simulink model "Test_Schnittstelle"  (R2018a)
settings: Solver=FixedStepAuto  StartTime=0.0  StopTime=inf  FixedStep=0.0000001  RelTol=1e-3
model workspace (MAT data in the model file):
  Address = Simulink.Signal
  Address.DataType = 'double'
  Address.Dimensions = 1
  Address.DimensionsMode = 'Fixed'
  Address.Complexity = 'real'
  Address.SampleTime = -1
  Address.SamplingMode = 'auto'
  Address.InitialValue = '0'
  De_1 = Simulink.Signal
  De_1.DataType = 'double'
  De_1.Dimensions = 1
  De_1.DimensionsMode = 'Fixed'
  De_1.Complexity = 'real'
  De_1.SampleTime = -1
  De_1.SamplingMode = 'auto'
  De_1.InitialValue = '0'
  De_2 = Simulink.Signal
  De_2.DataType = 'double'
  De_2.Dimensions = 1
  De_2.DimensionsMode = 'Fixed'
  De_2.Complexity = 'real'
  De_2.SampleTime = -1
  De_2.SamplingMode = 'auto'
  De_sum_1 = Simulink.Signal
  De_sum_1.DataType = 'double'
  De_sum_1.Dimensions = -1
  De_sum_1.DimensionsMode = 'Fixed'
  De_sum_1.Complexity = 'real'
  De_sum_1.SampleTime = -1
  De_sum_1.SamplingMode = 'auto'
  De_sum_1.InitialValue = '0'
  De_sum_2 = Simulink.Signal
  De_sum_2.DataType = 'double'
  De_sum_2.Dimensions = -1
  De_sum_2.DimensionsMode = 'Fixed'
  De_sum_2.Complexity = 'real'
  De_sum_2.SampleTime = -1
  De_sum_2.SamplingMode = 'auto'
  De_sum_2.InitialValue = '0'
  Filter = Simulink.Signal
  Filter.DataType = 'double'
  Filter.Dimensions = [20 7]
  Filter.DimensionsMode = 'Fixed'
  Filter.Complexity = 'real'
  Filter.SampleTime = -1
  Filter.SamplingMode = 'auto'
  Filter.InitialValue = 'zeros(20,7)'
  Handshake_1 = Simulink.Signal
  Handshake_1.DataType = 'boolean'
  Handshake_1.Dimensions = -1
  Handshake_1.DimensionsMode = 'Fixed'
  Handshake_1.Complexity = 'real'
  Handshake_1.SampleTime = -1
  Handshake_1.SamplingMode = 'auto'
  Handshake_1.InitialValue = 'false'
  Handshake_2 = Simulink.Signal
  Handshake_2.DataType = 'boolean'
  Handshake_2.Dimensions = -1
  Handshake_2.DimensionsMode = 'Fixed'
  Handshake_2.Complexity = 'real'
  Handshake_2.SampleTime = -1
  Handshake_2.SamplingMode = 'auto'
  Handshake_2.InitialValue = 'false'
  Recv_Buffer = Simulink.Signal
  Recv_Buffer.DataType = 'double'
  Recv_Buffer.Dimensions = [20 7]
  Recv_Buffer.DimensionsMode = 'Fixed'
  Recv_Buffer.Complexity = 'real'
  Recv_Buffer.SampleTime = -1
  Recv_Buffer.SamplingMode = 'auto'
  Recv_Buffer.InitialValue = 'zeros(20,7)'
  Send_Buffer_1 = Simulink.Signal
  Send_Buffer_1.DataType = 'double'
  Send_Buffer_1.Dimensions = [1 100]
  Send_Buffer_1.DimensionsMode = 'Fixed'
  Send_Buffer_1.Complexity = 'real'
  Send_Buffer_1.SampleTime = -1
  Send_Buffer_1.SamplingMode = 'auto'
  Send_Buffer_1.InitialValue = '[101, 102, zeros(1,98)]'
  Send_Buffer_2 = Simulink.Signal
  Send_Buffer_2.DataType = 'double'
  Send_Buffer_2.Dimensions = [1 100]
  Send_Buffer_2.DimensionsMode = 'Fixed'
  Send_Buffer_2.Complexity = 'real'
  Send_Buffer_2.SampleTime = -1
  Send_Buffer_2.SamplingMode = 'auto'
  Send_Buffer_2.InitialValue = '[101, 102, zeros(1,98)]'
  T_recv_1 = Simulink.Signal
  T_recv_1.DataType = 'double'
  T_recv_1.Dimensions = 1
  T_recv_1.DimensionsMode = 'Fixed'
  T_recv_1.Complexity = 'real'
  T_recv_1.SampleTime = -1
  T_recv_1.SamplingMode = 'auto'
  T_recv_1.InitialValue = '0'
  T_recv_2 = Simulink.Signal
  T_recv_2.DataType = 'auto'
  T_recv_2.Dimensions = 1
  T_recv_2.DimensionsMode = 'Fixed'
  T_recv_2.Complexity = 'real'
  T_recv_2.SampleTime = -1
  T_recv_2.SamplingMode = 'auto'
  T_recv_2.InitialValue = '0'
  T_send_1 = Simulink.Signal
  T_send_1.DataType = 'double'
  T_send_1.Dimensions = 1
  T_send_1.DimensionsMode = 'Fixed'
  T_send_1.Complexity = 'real'
  T_send_1.SampleTime = -1
  T_send_1.SamplingMode = 'auto'
  T_send_1.InitialValue = '0'
  T_send_2 = Simulink.Signal
  T_send_2.DataType = 'double1'
  T_send_2.Dimensions = 1
  T_send_2.DimensionsMode = 'Fixed'
  T_send_2.Complexity = 'real'
  T_send_2.SampleTime = -1
  T_send_2.SamplingMode = 'auto'
(part 1 of 2)
settings Model: Creator=张紫薇  LastModifiedBy=lenovo

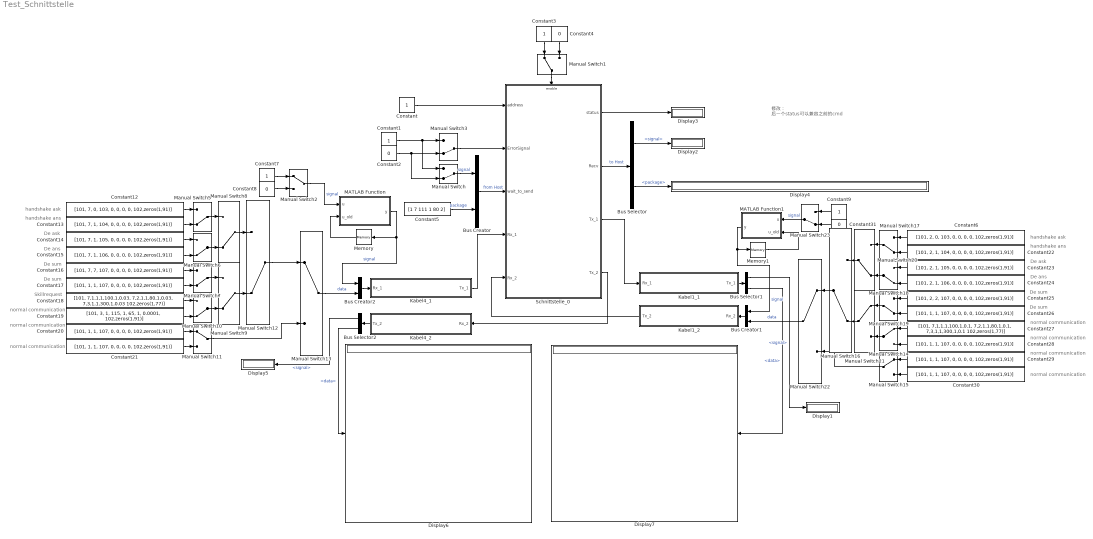
== system Test_Schnittstelle ==
  note: 修改：
      | 后一个status可以兼容之前的cmd
  note: handshake ask
  note: handshake ans
  note: De ask
  note: De ans
  note: De sum
  note: De sum
  note: Skillrequest
  note: normal communication
  note: normal communication
  note: normal communication
  note: normal communication
  note: normal communication
  note: handshake ask
  note: normal communication
  note: De sum
  note: handshake ans
  note: normal communication
  note: De ans
  note: De ask
  note: De sum
  Bus Creator : BusCreator  Inputs=2
  Bus Creator1 : BusCreator  Inputs=2
  Bus Creator2 : BusCreator  Inputs=2
  Bus Selector : BusSelector  OutputSignals=signal,package
  Bus Selector1 : BusSelector  OutputSignals=signal,data
  Bus Selector2 : BusSelector  OutputSignals=signal,data
  Constant : Constant  OutDataTypeStr=double
  Constant{1,3,7,9} (4 alike) : Constant  OutDataTypeStr=boolean
  Constant12 : Constant  Value=[101, 7, 0, 103, 0, 0, 0, 0, 102,zeros(1,91)]  OutDataTypeStr=double
  Constant13 : Constant  Value=[101, 7, 1, 104, 0, 0, 0, 0, 102,zeros(1,91)]  OutDataTypeStr=double
  Constant14 : Constant  Value=[101, 7, 1, 105, 0, 0, 0, 0, 102,zeros(1,91)]  OutDataTypeStr=double
  Constant15 : Constant  Value=[101, 7, 1, 106, 0, 0, 0, 0, 102,zeros(1,91)]  OutDataTypeStr=double
  Constant16 : Constant  Value=[101, 7, 7, 107, 0, 0, 0, 0, 102,zeros(1,91)]  OutDataTypeStr=double
  Constant{17,20..21,26,28..30} (7 alike) : Constant  Value=[101, 1, 1, 107, 0, 0, 0, 0, 102,zeros(1,91)]  OutDataTypeStr=double
  Constant18 : Constant  Value=[101, 7,1,1,1,100,1,0.03, 7,2,1,1,80,1,0.03, 7,3,1,1,300,1,0.03 102,zeros(1,77)]  OutDataTypeStr=double
  Constant19 : Constant  Value=[101, 3, 1, 115, 1, 65, 1, 0.0001, 102,zeros(1,91)]  OutDataTypeStr=double
  Constant{2,4,8,31} (4 alike) : Constant  Value=0  OutDataTypeStr=boolean
  Constant22 : Constant  Value=[101, 2, 1, 104, 0, 0, 0, 0, 102,zeros(1,91)]  OutDataTypeStr=double
  Constant23 : Constant  Value=[101, 2, 1, 105, 0, 0, 0, 0, 102,zeros(1,91)]  OutDataTypeStr=double
  Constant24 : Constant  Value=[101, 2, 1, 106, 0, 0, 0, 0, 102,zeros(1,91)]  OutDataTypeStr=double
  Constant25 : Constant  Value=[101, 2, 2, 107, 0, 0, 0, 0, 102,zeros(1,91)]  OutDataTypeStr=double
  Constant27 : Constant  Value=[101, 7,1,1,1,100,1,0.1, 7,2,1,1,80,1,0.1, 7,3,1,1,300,1,0.1 102,zeros(1,77)]  OutDataTypeStr=double
  Constant5 : Constant  Value=[1 7 111 1 80 2]  OutDataTypeStr=double
  Constant6 : Constant  Value=[101, 2, 0, 103, 0, 0, 0, 0, 102,zeros(1,91)]  OutDataTypeStr=double
  Display{1..7} (7 alike) : Display
      Display4 settings: Decimation=7
  Kabel1_1 : Subsystem  TreatAsAtomicUnit=on
  Kabel1_2 : Subsystem  TreatAsAtomicUnit=on
  Kabel4_1 : Subsystem  TreatAsAtomicUnit=on
  Kabel4_2 : Subsystem  TreatAsAtomicUnit=on
  MATLAB Function : MATLAB Function  TreatAsAtomicUnit=on  SystemSampleTime=0.00001
  MATLAB Function1 : MATLAB Function  TreatAsAtomicUnit=on  SystemSampleTime=0.00001
  Manual Switch{,3,5..10,12,16..20,23} (15 alike) : ManualSwitch  CurrentSetting=0
  Manual Switch{1..2,11,13..15,21..22} (8 alike) : ManualSwitch
  Memory : Memory  InitialCondition=false
  Memory1 : Memory  InitialCondition=false
  Schnittstelle_0 : Subsystem
  wires:
  Kabel4_2/1(Tx_2) -> Bus Selector2/1
  Bus Creator1/1 -> Kabel1_2/1(Rx_2)
  Bus Selector2/1 -> Display5/1  "<signal>"
  Bus Creator/1 -> Schnittstelle_0/3(wait_to_send)  "from Host"
  Constant8/1 -> Manual Switch2/2
  Kabel4_1/1(Tx_1) -> Schnittstelle_0/4(Rx_1)
  Manual Switch/1 -> Bus Creator/1  "signal"
  Bus Selector/1 -> Display2/1  "<signal>"
  Kabel1_1/1(Tx_1) -> Bus Selector1/1
  Manual Switch3/1 -> Schnittstelle_0/2(ErrorSignal)
  Bus Selector/2 -> Display4/1  "<package>"
  Manual Switch13/1 -> Bus Creator2/2  "data"
  MATLAB Function/1(y) -> Bus Creator2/1, Memory/1  "signal"
  Constant5/1 -> Bus Creator/2  "package"
  Constant7/1 -> Manual Switch2/1
  Kabel1_2/1(Tx_2) -> Schnittstelle_0/5(Rx_2)
  Constant4/1 -> Manual Switch1/2
  Constant1/1 -> Manual Switch/1, Manual Switch3/1
  Constant3/1 -> Manual Switch1/1
  Constant/1 -> Schnittstelle_0/1(address)
  MATLAB Function1/1(y) -> Bus Creator1/1, Memory1/1  "signal"
  Bus Selector1/1 -> Display1/1  "<signal>"
  Bus Creator2/1 -> Kabel4_1/1(Rx_1)
  Schnittstelle_0/1(status) -> Display3/1
  Bus Selector1/2 -> Display7/1  "<data>"
  Schnittstelle_0/4(Tx_2) -> Kabel4_2/1(Rx_2)
  Manual Switch1/1 -> Schnittstelle_0/Enable
  Constant2/1 -> Manual Switch/2, Manual Switch3/2
  Bus Selector2/2 -> Display6/1  "<data>"
  Schnittstelle_0/2(Recv) -> Bus Selector/1  "to Host"
  Schnittstelle_0/3(Tx_1) -> Kabel1_1/1(Rx_1)
  Constant12/1 -> Manual Switch5/1
  Constant13/1 -> Manual Switch5/2
  Constant14/1 -> Manual Switch6/1
  Constant15/1 -> Manual Switch6/2
  Constant16/1 -> Manual Switch7/1
  Constant17/1 -> Manual Switch7/2
  Manual Switch5/1 -> Manual Switch8/1
  Manual Switch6/1 -> Manual Switch8/2
  Manual Switch7/1 -> Manual Switch9/1
  Manual Switch10/1 -> Manual Switch9/2
  Constant18/1 -> Manual Switch10/1
  Constant19/1 -> Manual Switch10/2
  Constant20/1 -> Manual Switch11/1
  Constant21/1 -> Manual Switch11/2
  Manual Switch9/1 -> Manual Switch12/2
  Manual Switch8/1 -> Manual Switch12/1
  Manual Switch12/1 -> Manual Switch13/1
  Manual Switch11/1 -> Manual Switch13/2
  Constant6/1 -> Manual Switch17/1
  Constant22/1 -> Manual Switch17/2
  Constant23/1 -> Manual Switch18/1
  Constant24/1 -> Manual Switch18/2
  Constant25/1 -> Manual Switch19/1
  Constant26/1 -> Manual Switch19/2
  Constant27/1 -> Manual Switch14/1
  Constant28/1 -> Manual Switch14/2
  Constant29/1 -> Manual Switch15/1
  Constant30/1 -> Manual Switch15/2
  Manual Switch17/1 -> Manual Switch20/1
  Manual Switch18/1 -> Manual Switch20/2
  Manual Switch19/1 -> Manual Switch21/1
  Manual Switch14/1 -> Manual Switch21/2
  Manual Switch20/1 -> Manual Switch16/1
  Manual Switch21/1 -> Manual Switch16/2
  Manual Switch15/1 -> Manual Switch22/2
  Manual Switch22/1 -> Bus Creator1/2  "data"
  Manual Switch16/1 -> Manual Switch22/1
  Manual Switch2/1 -> MATLAB Function/1(u)  "signal"
  Memory/1 -> MATLAB Function/2(u_old)
  Memory1/1 -> MATLAB Function1/2(u_old)
  Manual Switch23/1 -> MATLAB Function1/1(u)  "signal"
  Constant9/1 -> Manual Switch23/1
  Constant31/1 -> Manual Switch23/2

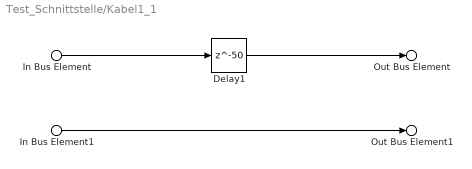
== system Test_Schnittstelle/Kabel1_1 ==
  In Bus Element : Inport  PortName=Rx_1  Element=signal
  In Bus Element1 : Inport  PortName=Rx_1  Element=data
  Delay1 : Delay  DelayLength=50
  Out Bus Element : Outport  PortName=Tx_1  Element=signal
  Out Bus Element1 : Outport  PortName=Tx_1  Element=data
  wires:
  In Bus Element/1 -> Delay1/1
  Delay1/1 -> Out Bus Element/1
  In Bus Element1/1 -> Out Bus Element1/1

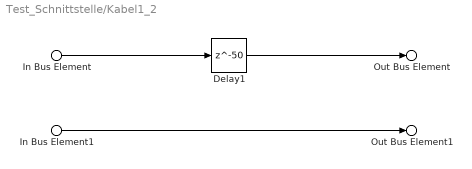
== system Test_Schnittstelle/Kabel1_2 ==
  In Bus Element : Inport  PortName=Rx_2  Element=signal
  In Bus Element1 : Inport  PortName=Rx_2  Element=data
  Delay1 : Delay  DelayLength=50
  Out Bus Element : Outport  PortName=Tx_2  Element=signal
  Out Bus Element1 : Outport  PortName=Tx_2  Element=data
  wires:
  In Bus Element/1 -> Delay1/1
  Delay1/1 -> Out Bus Element/1
  In Bus Element1/1 -> Out Bus Element1/1

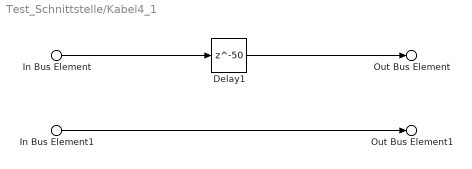
== system Test_Schnittstelle/Kabel4_1 ==
  In Bus Element : Inport  PortName=Rx_1  Element=signal
  In Bus Element1 : Inport  PortName=Rx_1  Element=data
  Delay1 : Delay  DelayLength=50
  Out Bus Element : Outport  PortName=Tx_1  Element=signal
  Out Bus Element1 : Outport  PortName=Tx_1  Element=data
  wires:
  In Bus Element/1 -> Delay1/1
  Delay1/1 -> Out Bus Element/1
  In Bus Element1/1 -> Out Bus Element1/1

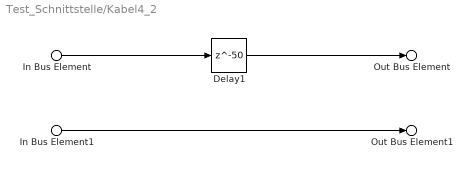
== system Test_Schnittstelle/Kabel4_2 ==
  In Bus Element : Inport  PortName=Rx_2  Element=signal
  In Bus Element1 : Inport  PortName=Rx_2  Element=data
  Delay1 : Delay  DelayLength=50
  Out Bus Element : Outport  PortName=Tx_2  Element=signal
  Out Bus Element1 : Outport  PortName=Tx_2  Element=data
  wires:
  In Bus Element/1 -> Delay1/1
  Delay1/1 -> Out Bus Element/1
  In Bus Element1/1 -> Out Bus Element1/1

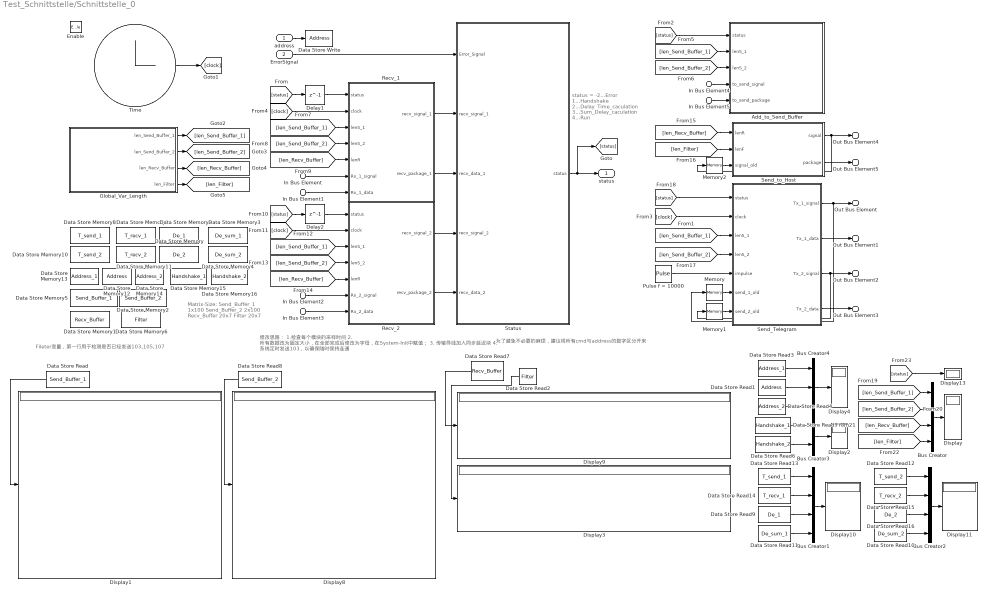
== system Test_Schnittstelle/Schnittstelle_0 ==
  note: 为了避免不必要的麻烦，建议将所有cmd与address的数字区分开来
  note: Fileter变量，第一行用于检测是否已经发送103,105,107
  note: 修改思路：
      | 1.检查每个模块的采样时间
      | 2. 所有数据改为固定大小，在全部完成后修改为字母，在System-Init中赋值；
      | 3. 传输导线加入同步延迟块
      | 4. 系统定时发送103，以确保随时保持连通
  note: status =
      | -2...Error
      |  1...Handshake
      |  2...Delay_Time_caculation
      |  3...Sum_Delay_caculation
      |  4...Run
  note: Matrix-Size:
      | Send_Buffer_1	1x100
      | Send_Buffer_2	2x100
      | Recv_Buffer		20x7
      | Filter			20x7
  address : Inport
  ErrorSignal : Inport  Port=2
  In Bus Element4 : Inport  Port=3  PortName=wait_to_send  Element=signal
  In Bus Element5 : Inport  Port=3  PortName=wait_to_send  Element=package
  In Bus Element : Inport  Port=4  PortName=Rx_1  Element=signal
  In Bus Element1 : Inport  Port=4  PortName=Rx_1  Element=data
  In Bus Element2 : Inport  Port=5  PortName=Rx_2  Element=signal
  In Bus Element3 : Inport  Port=5  PortName=Rx_2  Element=data
  Enable : EnablePort
  Add_to_Send_Buffer : MATLAB Function  TreatAsAtomicUnit=on  SystemSampleTime=0.00001
  Bus Creator : BusCreator  Inputs=4
  Bus Creator1 : BusCreator  Inputs=4
  Bus Creator2 : BusCreator  Inputs=4
  Bus Creator3 : BusCreator  Inputs=2
  Bus Creator4 : BusCreator  Inputs=3
  Data Store Memory : DataStoreMemory  DataStoreName=De_2  ReadBeforeWriteMsg=warning  WriteAfterWriteMsg=warning  WriteAfterReadMsg=warning  ShowAdditionalParam=off  OutDataTypeStr=double  Dimensions=1
  Data Store Memory1 : DataStoreMemory  DataStoreName=Recv_Buffer  ReadBeforeWriteMsg=warning  WriteAfterWriteMsg=warning  WriteAfterReadMsg=warning  InitialValue=zeros(20,7)  VectorParams1D=off  ShowAdditionalParam=off  OutDataTypeStr=double  Dimensions=[20,7]
  Data Store Memory10 : DataStoreMemory  DataStoreName=T_send_2  ReadBeforeWriteMsg=warning  WriteAfterWriteMsg=warning  WriteAfterReadMsg=warning  ShowAdditionalParam=off  OutDataTypeStr=double  Dimensions=1
  Data Store Memory11 : DataStoreMemory  DataStoreName=T_recv_2  ReadBeforeWriteMsg=warning  WriteAfterWriteMsg=warning  WriteAfterReadMsg=warning  ShowAdditionalParam=off  OutDataTypeStr=double  Dimensions=1
  Data Store Memory12 : DataStoreMemory  DataStoreName=Address  ReadBeforeWriteMsg=warning  WriteAfterWriteMsg=warning  WriteAfterReadMsg=warning  ShowAdditionalParam=off  OutDataTypeStr=double  Dimensions=1
  Data Store Memory13 : DataStoreMemory  DataStoreName=Address_1  ReadBeforeWriteMsg=warning  WriteAfterWriteMsg=warning  WriteAfterReadMsg=warning  ShowAdditionalParam=off  OutDataTypeStr=double  Dimensions=1
  Data Store Memory14 : DataStoreMemory  DataStoreName=Address_2  ReadBeforeWriteMsg=warning  WriteAfterWriteMsg=warning  WriteAfterReadMsg=warning  ShowAdditionalParam=off  OutDataTypeStr=double  Dimensions=1
  Data Store Memory15 : DataStoreMemory  DataStoreName=Handshake_1  ReadBeforeWriteMsg=warning  WriteAfterWriteMsg=warning  WriteAfterReadMsg=warning  InitialValue=false  ShowAdditionalParam=off  OutDataTypeStr=boolean
  Data Store Memory16 : DataStoreMemory  DataStoreName=Handshake_2  ReadBeforeWriteMsg=warning  WriteAfterWriteMsg=warning  WriteAfterReadMsg=warning  InitialValue=false  ShowAdditionalParam=off  OutDataTypeStr=boolean
  Data Store Memory2 : DataStoreMemory  DataStoreName=Send_Buffer_2  ReadBeforeWriteMsg=warning  WriteAfterWriteMsg=warning  WriteAfterReadMsg=warning  InitialValue=[101, 102, zeros(1,98)]  VectorParams1D=off  ShowAdditionalParam=off  OutDataTypeStr=double  Dimensions=[1,100]
  Data Store Memory3 : DataStoreMemory  DataStoreName=De_sum_1  ReadBeforeWriteMsg=warning  WriteAfterWriteMsg=warning  WriteAfterReadMsg=warning  ShowAdditionalParam=off  OutDataTypeStr=double  Dimensions=1
  Data Store Memory4 : DataStoreMemory  DataStoreName=De_sum_2  ReadBeforeWriteMsg=warning  WriteAfterWriteMsg=warning  WriteAfterReadMsg=warning  ShowAdditionalParam=off  OutDataTypeStr=double  Dimensions=1
  Data Store Memory5 : DataStoreMemory  DataStoreName=Send_Buffer_1  ReadBeforeWriteMsg=warning  WriteAfterWriteMsg=warning  WriteAfterReadMsg=warning  InitialValue=[101, 102, zeros(1,98)]  VectorParams1D=off  ShowAdditionalParam=off  OutDataTypeStr=double  Dimensions=[1,100]
  Data Store Memory6 : DataStoreMemory  DataStoreName=Filter  ReadBeforeWriteMsg=warning  WriteAfterWriteMsg=warning  WriteAfterReadMsg=warning  InitialValue=zeros(20,7)  VectorParams1D=off  ShowAdditionalParam=off  OutDataTypeStr=double  Dimensions=[20,7]
  Data Store Memory7 : DataStoreMemory  DataStoreName=De_1  ReadBeforeWriteMsg=warning  WriteAfterWriteMsg=warning  WriteAfterReadMsg=warning  ShowAdditionalParam=off  OutDataTypeStr=double  Dimensions=1
  Data Store Memory8 : DataStoreMemory  DataStoreName=T_send_1  ReadBeforeWriteMsg=warning  WriteAfterWriteMsg=warning  WriteAfterReadMsg=warning  ShowAdditionalParam=off  OutDataTypeStr=double  Dimensions=1
  Data Store Memory9 : DataStoreMemory  DataStoreName=T_recv_1  ReadBeforeWriteMsg=warning  WriteAfterWriteMsg=warning  WriteAfterReadMsg=warning  ShowAdditionalParam=off  OutDataTypeStr=double  Dimensions=1
  Data Store Read : DataStoreRead  DataStoreName=Send_Buffer_1
  Data Store Read1 : DataStoreRead  DataStoreName=Address
  Data Store Read10 : DataStoreRead  DataStoreName=De_sum_2
  Data Store Read11 : DataStoreRead  DataStoreName=De_sum_1
  Data Store Read12 : DataStoreRead  DataStoreName=T_send_2
  Data Store Read13 : DataStoreRead  DataStoreName=T_send_1
  Data Store Read14 : DataStoreRead  DataStoreName=T_recv_1
  Data Store Read15 : DataStoreRead  DataStoreName=T_recv_2
  Data Store Read16 : DataStoreRead  DataStoreName=De_2
  Data Store Read2 : DataStoreRead  DataStoreName=Filter
  Data Store Read3 : DataStoreRead  DataStoreName=Address_1
  Data Store Read4 : DataStoreRead  DataStoreName=Address_2
  Data Store Read5 : DataStoreRead  DataStoreName=Handshake_1
  Data Store Read6 : DataStoreRead  DataStoreName=Handshake_2
  Data Store Read7 : DataStoreRead  DataStoreName=Recv_Buffer
  Data Store Read8 : DataStoreRead  DataStoreName=Send_Buffer_2
  Data Store Read9 : DataStoreRead  DataStoreName=De_1
  Data Store Write : DataStoreWrite  DataStoreName=Address
  Delay1 : Delay  DelayLength=1
  Delay2 : Delay  DelayLength=1
  Display{,1..4,8..11,13} (10 alike) : Display
  Global_Var_Length : MATLAB Function  TreatAsAtomicUnit=on
  Memory : Memory  InitialCondition=false
  Memory1 : Memory  InitialCondition=false
  Memory2 : Memory  InitialCondition=false
  Pulse f = 10000 : DiscretePulseGenerator  PulseType=Time based  Amplitude=true  Period=1/1000  PulseWidth=30
  Recv_1 : MATLAB Function  TreatAsAtomicUnit=on  SystemSampleTime=0.00001
  Recv_2 : MATLAB Function  TreatAsAtomicUnit=on  SystemSampleTime=0.00001
  Send_Telegram : MATLAB Function  TreatAsAtomicUnit=on  SystemSampleTime=0.00001
  Send_to_Host : MATLAB Function  TreatAsAtomicUnit=on  SystemSampleTime=0.00001
  Status : Stateflow chart  TreatAsAtomicUnit=on  SystemSampleTime=0.0000001
  Time : Clock
  status : Outport
  Out Bus Element4 : Outport  Port=2  PortName=Recv  Element=signal
  Out Bus Element5 : Outport  Port=2  PortName=Recv  Element=package
  Out Bus Element : Outport  Port=3  PortName=Tx_1  Element=signal
  Out Bus Element1 : Outport  Port=3  PortName=Tx_1  Element=data
  Out Bus Element2 : Outport  Port=4  PortName=Tx_2  Element=signal
  Out Bus Element3 : Outport  Port=4  PortName=Tx_2  Element=data
  wires:
  ErrorSignal/1 -> Status/1(Error_Signal)
  Status/1(status) -> [status], status/1
  Pulse f = 10000/1 -> Send_Telegram/5(impulse)
  In Bus Element1/1 -> Recv_1/7(Rx_1_data)
  In Bus Element/1 -> Recv_1/6(Rx_1_signal)
  Send_Telegram/1(Tx_1_signal) -> Memory/1, Out Bus Element/1
  Send_Telegram/3(Tx_2_signal) -> Memory1/1, Out Bus Element2/1
  Memory1/1 -> Send_Telegram/7(send_2_old)
  Memory/1 -> Send_Telegram/6(send_1_old)
  [status] -> Delay1/1
  Time/1 -> [clock]
  [clock] -> Recv_1/2(clock)
  Send_to_Host/1(signal) -> Out Bus Element4/1, Memory2/1
  address/1 -> Data Store Write/1
  Global_Var_Length/1(len_Send_Buffer_1) -> [len_Send_Buffer_1]
  Global_Var_Length/2(len_Send_Buffer_2) -> [len_Send_Buffer_2]
  Global_Var_Length/3(len_Recv_Buffer) -> [len_Recv_Buffer]
  Global_Var_Length/4(len_Filter) -> [len_Filter]
  [len_Send_Buffer_1] -> Recv_1/3(lenS_1)
  [len_Send_Buffer_2] -> Recv_1/4(lenS_2)
  [len_Recv_Buffer] -> Recv_1/5(lenR)
  In Bus Element2/1 -> Recv_2/6(Rx_2_signal)
  In Bus Element3/1 -> Recv_2/7(Rx_2_data)
  [status] -> Delay2/1
  [len_Recv_Buffer] -> Recv_2/5(lenR)
  [len_Send_Buffer_1] -> Recv_2/3(lenS_1)
  [clock] -> Recv_2/2(clock)
  [len_Send_Buffer_2] -> Recv_2/4(lenS_2)
  Delay1/1 -> Recv_1/1(status)
  Delay2/1 -> Recv_2/1(status)
  Recv_1/1(recv_signal_1) -> Status/2(recv_signal_1)
  Recv_1/2(recv_package_1) -> Status/3(recv_data_1)
  Recv_2/1(recv_signal_2) -> Status/4(recv_signal_2)
  Recv_2/2(recv_package_2) -> Status/5(recv_data_2)
  [len_Recv_Buffer] -> Send_to_Host/1(lenR)
  [len_Filter] -> Send_to_Host/2(lenF)
  Send_Telegram/4(Tx_2_data) -> Out Bus Element3/1
  [len_Send_Buffer_1] -> Send_Telegram/3(lenS_1)
  [len_Send_Buffer_2] -> Send_Telegram/4(lenS_2)
  [clock] -> Send_Telegram/2(clock)
  [status] -> Send_Telegram/1(status)
  Send_Telegram/2(Tx_1_data) -> Out Bus Element1/1
  [len_Send_Buffer_1] -> Add_to_Send_Buffer/2(lenS_1)
  [len_Send_Buffer_2] -> Add_to_Send_Buffer/3(lenS_2)
  In Bus Element4/1 -> Add_to_Send_Buffer/4(to_send_signal)
  In Bus Element5/1 -> Add_to_Send_Buffer/5(to_send_package)
  [status] -> Add_to_Send_Buffer/1(status)
  Memory2/1 -> Send_to_Host/3(signal_old)
  Bus Creator/1 -> Display/1
  [len_Send_Buffer_1] -> Bus Creator/1
  [len_Send_Buffer_2] -> Bus Creator/2
  [len_Recv_Buffer] -> Bus Creator/3
  [len_Filter] -> Bus Creator/4
  Data Store Read/1 -> Display1/1
  Data Store Read2/1 -> Display3/1
  Data Store Read8/1 -> Display8/1
  Data Store Read7/1 -> Display9/1
  Data Store Read13/1 -> Bus Creator1/1
  Data Store Read14/1 -> Bus Creator1/2
  Data Store Read11/1 -> Bus Creator1/4
  Data Store Read9/1 -> Bus Creator1/3
  Bus Creator1/1 -> Display10/1
  Data Store Read12/1 -> Bus Creator2/1
  Data Store Read15/1 -> Bus Creator2/2
  Bus Creator2/1 -> Display11/1
  Data Store Read16/1 -> Bus Creator2/3
  Data Store Read10/1 -> Bus Creator2/4
  [status] -> Display13/1
  Send_to_Host/2(package) -> Out Bus Element5/1
  Data Store Read5/1 -> Bus Creator3/1
  Data Store Read6/1 -> Bus Creator3/2
  Data Store Read4/1 -> Bus Creator4/3
  Data Store Read1/1 -> Bus Creator4/2
  Data Store Read3/1 -> Bus Creator4/1
  Bus Creator3/1 -> Display2/1
  Bus Creator4/1 -> Display4/1

== matlab function Test_Schnittstelle/Schnittstelle_0/Add_to_Send_Buffer ==
  data: Send_Buffer_1 data_store_memory; Send_Buffer_2 data_store_memory; Address data_store_memory; status input; lenS_1 input; lenS_2 input; to_send_signal input; to_send_package input; Address_1 data_store_memory; Address_2 data_store_memory; Handshake_1 data_store_memory; Handshake_2 data_store_memory; Filter data_store_memory; De_1 data_store_memory; De_2 data_store_memory; De_sum_1 data_store_memory; De_sum_2 data_store_memory
% Name: add_to_Send_Buffer
% Funktionalitäten
% Handshake-Message einfügen, wenn Status==1
% Delay-caculation-Message einfügen, wenn Status==2
% Sum-Delay-caculation-Message einfügen, wemm Status==3
% Nachrichten, die der Host senden möchte, einfügen, wenn Status==4

function add_to_Send_Buffer(status, lenS_1, lenS_2, to_send_signal, to_send_package)

global Send_Buffer_1
global Send_Buffer_2
global Address
global Address_1
global Address_2
global Handshake_1
global Handshake_2
global Filter
global De_1
global De_2
global De_sum_1
global De_sum_2

switch status
    case -2                         % Error Signal einrichten
        Filter(1,7) = 1;
    case 1                          % Handshake
        if((Filter(1,1) == 0) || ~Handshake_1)              % 103 not sent yet || Handshake_1 not finish yet
            check_1 = check_X(103, Address, Send_Buffer_1);          % check if there is a 103-Message in Send_Buffer_1
            if ~check_1
                Send_Buffer_1(lenS_1:lenS_1+7) = [Address, 0, 103, zeros(1,4), 102];
                Filter(1,1) = 1;                            % to remember, if 103 ist sent
            end
        end
        if((Filter(1,2) == 0) || ~Handshake_2)
            check_2 = check_X(103, Address, Send_Buffer_2);
            if ~check_2
                Send_Buffer_2(lenS_2:lenS_2+7) = [Address, 0, 103, zeros(1,4), 102];
                Filter(1,2) = 1;
            end
        end

        
    case 2                          % Delay time caculation
        if((Filter(1,3) == 0 ) || (De_1 <= 0))              % 105 not sent || De_1 not caculated yet
            check_1 = check_X(105, Address, Send_Buffer_1);
            if ~check_1
                Send_Buffer_1(lenS_1:lenS_1+7) = [Address, Address_2, 105, zeros(1,4), 102];
                Filter(1,3) = 1;
            end
        end
        if((Filter(1,4) == 0 ) || (De_2 <= 0))
            check_2 = check_X(105, Address, Send_Buffer_2);
            if ~check_2
                Send_Buffer_2(lenS_2:lenS_2+7) = [Address, Address_1, 105, zeros(1,4), 102];
                Filter(1,4) = 1;
            end
        end
        
    case 3                          % Sum_Delay caculation
        if((Filter(1,5) == 0 ) || (De_sum_1 <= 0))          % 107 not sent || De_sum_1 not caculated yet
            check_1 = check_X(107, Address, Send_Buffer_1);
            if ~check_1
                Send_Buffer_1(lenS_1:lenS_1+7) = [Address, Address, 107, zeros(1,4), 102];
                Filter(1,5) = 1;
            end
        end
        if((Filter(1,6) == 0 ) || (De_sum_2 <= 0))
            check_2 = check_X(107, Address, Send_Buffer_2);
            if ~check_2
                Send_Buffer_2(lenS_2:lenS_2+7) = [Address, Address, 107, zeros(1,4), 102];
                Filter(1,6) = 1;
            end
        end
        
    case 4                          % normal communication
        if to_send_signal
            check_1 = check_Y(to_send_package, Send_Buffer_1);
            check_2 = check_Y(to_send_package, Send_Buffer_2);
            if ~check_1
                Send_Buffer_1(lenS_1:lenS_1+7) = [to_send_package', 0, 102];
            end
            if ~check_2
                Send_Buffer_2(lenS_2:lenS_2+7) = [to_send_package', 0, 102];
            end
        end
end

end

function y = check_X(CMD, adr, Data)          % y: boolean; x: double, [1x100];

x = find(Data==CMD);
y = ~isempty(x);
if y
    y = y && (Data(1,x(1)-2) == adr);
end

end

function y = check_Y(data, Data)          % y: boolean; data: double, [1x6];

x = find(Data==data(3));        % CMD
y = ~isempty(x);
if y
    for i=1:length(x)
        if(isequal(Data(x(i)-2:x(i)+3),data'))
            y = true;
            break
        else
            y = false;
        end
    end
end

end

== matlab function Test_Schnittstelle/Schnittstelle_0/Send_Telegram ==
  data: status input double size=1; clock input double; lenS_1 input; lenS_2 input; impulse input boolean size=1; Tx_1_signal output boolean size=1; Tx_1_data output double size=[1,100]; Tx_2_signal output; send_1_old input boolean size=1; send_2_old input boolean size=1; T_send_1 data_store_memory; T_send_2 data_store_memory; Tx_2_data output double size=[1,100]; Send_Buffer_1 data_store_memory; Send_Buffer_2 data_store_memory; De_1 data_store_memory; De_2 data_store_memory; De_sum_1 data_store_memory; De_sum_2 data_store_memory; Address data_store_memory
% Name: send_telegram
% Funktionalität:
% Datenpacket in Send_Buffer_1 und Send_Buffer2 zyklisch transferieren.
% Die Zykluszeit lautet 10ms

function [Tx_1_signal, Tx_1_data, Tx_2_signal, Tx_2_data] = send_telegram(status, clock, lenS_1, lenS_2, impulse, send_1_old, send_2_old)

global Send_Buffer_1
global Send_Buffer_2
global De_1
global De_2
global De_sum_1
global De_sum_2
global T_send_1
global T_send_2
global Address

timer_1 = 0;
timer_2 = 0;

if send_1_old || send_2_old
    % The Send_Signal lasts for only one period. Then it need to be shut down.
    Tx_1_signal = false;
	Tx_2_signal = false;
    Tx_1_data = zeros(1,100);
    Tx_2_data = zeros(1,100);
else
    % No Error + send-signal already shut down + Impulse-Signal --> OK! Let's send the telegram!
    if ((status > 0) && (~send_1_old) && (~send_2_old) && impulse)
        h1 = ceil((lenS_1 - 2) / 7);
        h2 = ceil((lenS_2 - 2) / 7);
        % Before send, we need check if we need to do something else. For example: 'start the Timer' or 'caculate a new De in each datablock'
        switch status
            case 2                                              % Delay time caculation
                if ~isempty(find(Send_Buffer_1==105,1))                     % check if there is a 105-cmd in Send_Buffer,if so, timer need to be started
                    timer_1 = 1;
                end
                if ~isempty(find(Send_Buffer_2==105,1))
                    timer_2 = 1;
                end

            case 3                                              % Sum_Delay caculation
                for i1=1:h1
                    if isequal([Send_Buffer_1(7*i1-5:7*i1-3),De_sum_1],[Address,Address,107,0])     % check if there is a 105-cmd in Send_Buffer
                        timer_1 = 1;
                        break
                    end
                end
                for i2=1:h2
                    if isequal([Send_Buffer_2(7*i2-5:7*i2-3),De_sum_2],[Address,Address,107,0])
    %                if ((Send_Buffer_2(7*i2-5) == Address) && (Send_Buffer_2(7*i2-4) == Address) && (Send_Buffer_2(7*i2-3) == 107) && De_sum_2 == 0)
                        timer_2 = 1;
                        break
                    end
                end

            case 4
                for i1=1:h1                                                    % recaculate the Delay time for each datablock
                    Send_Buffer_1(7*i1+1) = Send_Buffer_1(7*i1+1) + De_1;
                end
                for i2=1:h2
                    Send_Buffer_2(7*i2+1) = Send_Buffer_2(7*i2+1) + De_2;
                end
        end
        
        % Now we can send the telegram!!
        Tx_1_data = Send_Buffer_1;                                  % send data
        Tx_2_data = Send_Buffer_2;
        Tx_1_signal = true;
        Tx_2_signal = true;
        
        % remember the send-time if necessary
        if timer_1 == 1
            T_send_1 = clock;
        end
        if timer_2 == 1
            T_send_2 = clock;
        end
        % clear the data in Send_Buffer after sending
        if (lenS_1 > 2)
            Send_Buffer_1(1:lenS_1) = [101,102, zeros(1,lenS_1-2)];
        end
        if (lenS_2 > 2)
            Send_Buffer_2(1:lenS_2) = [101,102, zeros(1,lenS_2-2)];
        end
    else
        Tx_1_signal = false;
        Tx_1_data = zeros(1,100);
        Tx_2_signal = false;
        Tx_2_data = zeros(1,100);
    end
end

end

== matlab function Test_Schnittstelle/Schnittstelle_0/Recv_1 ==
  data: status input double size=1; clock input double size=1; lenS_1 input; lenS_2 input; lenR input; Rx_1_signal input boolean size=1; Rx_1_data input double size=[1 100]; recv_signal_1 output boolean; recv_package_1 output double size=[1 98]; Send_Buffer_1 data_store_memory; Send_Buffer_2 data_store_memory; T_send_1 data_store_memory; T_recv_1 data_store_memory; De_1 data_store_memory; De_sum_1 data_store_memory; Address data_store_memory; Recv_Buffer data_store_memory; Address_2 data_store_memory; Address_1 data_store_memory; De_sum_2 data_store_memory; Handshake_1 data_store_memory
% Name: Rx_1

% Funktionalitäten:
% Im Init-Prozess
%   1. Handshake durch zu führen
%       103...Handshake ask --> 104 in Send_Buffer_2 additieren
%       104...Handshake answer --> Handshake success
%   2. Delay-Zeit berechnen
%       105...Delay begin --> 106 in Send_Buffer_2 additieren
%       106...Delay end --> Delay_Zeit berechnen
%   3. Sum-Delay-Zeit berechnen
%       107, Receiver = meine Addresse --> Sum_Delay_Zeit berechnen
%       107, Receiver ~= meine Addresse --> Daten in Send_Buffer_1 additieren
% Im normalen Prozess
%   4. Receiver = meine Addresse --> in Recv_Buffer additieren
%   5. Receiver = 255 --> Broadcast --> in Recv_Buffer && Send_Buffer_1 additieren
%   6. Receiver ~= meine Addresse --> in Send_Buffer_1 additieren

function [recv_signal_1, recv_package_1] = Rx_1(status, clock,lenS_1, lenS_2, lenR, Rx_1_signal, Rx_1_data)

global Send_Buffer_1
global Send_Buffer_2
global T_send_1
global T_recv_1
global De_1
global De_sum_1
global Address
global Address_1
%global Address_2
global Recv_Buffer
global Handshake_1

recv_signal_1 = false;
recv_package_1 = zeros(1,98);       % one datablock = [1x7]

lenr = 1;                           % path to write data into recv_package_1

if Rx_1_signal
    a = find(Rx_1_data==102,1);
    len = a(1);
    if ~isempty(len)
        mod_ = mod(len-2,7);
        len_ = ceil((len - 2) / 7);                                 % Round toward positive infinity
    end
    
	if ((mod_ == 0) && (len_ >= 1))                             % package contains at least one datablock
        switch status
            case 1                                              % Handshake
                for i=1:len_
                    switch Rx_1_data(7*i-3)                          % Da.cmd
                        case 103                                % Handshake ask --> send answer
                            check = check_X(104, Address, Send_Buffer_2);
                            if ((Rx_1_data(7*i-5) ~= 0) && (Rx_1_data(7*i-4) == 0) && ~Handshake_1 && ~check)
                                Address_1 = Rx_1_data(7*i-5);
                                Send_Buffer_2(lenS_2:lenS_2+7) = [Address, Address_1, 104, zeros(1,4), 102];
                            end
                        case 104                                % Handshake answer --> Handshake success --> no more send
                            if ((Rx_1_data(7*i-5) ~= 0) && (Rx_1_data(7*i-4) == Address) && ~Handshake_1)
                                Address_1 = Rx_1_data(7*i-5);        % Address of the Host in the Direction_1
                                recv_package_1(lenr:lenr+6) = Rx_1_data(7*i-5:7*i+1);    % [_,_,104,_,_,_,_] = [1x7]
                                lenr = lenr + 7;
                                recv_signal_1 = true;
                            end
                    end
                end

            case 2                                              % Delay_Time_Caculation
                for j=1:len_
                    switch Rx_1_data(7*j-3)                          % Da.cmd
                        case 103                                % Handshake ask --> send answer
                            check = check_X(104, Address, Send_Buffer_2);
                            if ((Rx_1_data(7*j-5) ~= 0) && (Rx_1_data(7*j-4) == 0) && ~Handshake_1 && ~check)
                                Address_1 = Rx_1_data(7*j-5);
                                Send_Buffer_2(lenS_2:lenS_2+7) = [Address, Address_1, 104, zeros(1,4), 102];
                            end
                        case 105                                % Delay ask --> send answer
                            check = check_X(106, Address, Send_Buffer_2);
                            if (isequal(Rx_1_data(7*j-5:7*j-4),[Address_1, Address]) && Handshake_1 && ~check) % check Sender & Receiver
                                Send_Buffer_2(lenS_2:lenS_2+7) = [Address, 0, 106, zeros(1,4), 102];
                            end
                        case 106                                % Delay answer --> caculate the time --> no more send
                            if ((isequal(Rx_1_data(7*j-5:7*j-3),[Address_1, Address, 106])) && (De_1 <= 0))
                                T_recv_1 = clock;
                                De_1 = T_recv_1 - T_send_1;
                                T_send_1 = 0;
                                T_recv_1 = 0;
                            end
                    end
                end

            case 3                                              % Sum_Delay_Caculation
                for h=1:len_
                    switch Rx_1_data(7*h-3)
                        case 103                                % Handshake ask --> send answer
                            check = check_X(104, Address, Send_Buffer_2);
                            if ((Rx_1_data(7*h-5) ~= 0) && (Rx_1_data(7*h-4) == 0) && ~Handshake_1 && ~check)
                                Address_1 = Rx_1_data(7*h-5);
                                Send_Buffer_2(lenS_2:lenS_2+7) = [Address, Address_1, 104, zeros(1,4), 102];
                            end
                        case 105                                % Delay ask --> send answer
                            check = check_X(106, Address, Send_Buffer_2);
                            if (isequal(Rx_1_data(7*h-5:7*h-4),[Address_1, Address]) && Handshake_1 && ~check) % check Sender & Receiver
                                Send_Buffer_2(lenS_2:lenS_2+7) = [Address, 0, 106, zeros(1,4), 102];
                            end   
                        case 107
                            if (isequal(Rx_1_data(7*h-5:7*h-4),[Address, Address]) && (De_sum_1 <= De_1))                   % Sum_Delay --> caculate the time --> no more send
                                T_recv_1 = clock;
                                De_sum_1 = T_recv_1 - T_send_1;
                                T_send_1 = 0;
                                T_recv_1 = 0;
                            elseif ((isequal(Rx_1_data(7*h-5),Rx_1_data(7*h-4))) && (Rx_1_data(7*h-5) ~= Address))
                                check = check_Y(Rx_1_data(7*h-5:7*h), recv_package_1) && check_Y(Rx_1_data(7*h-5:7*h), Send_Buffer_1);
                                if ~check
                                    recv_package_1(lenr:lenr+6) = Rx_1_data(7*h-5:7*h+1)';
                                    lenr = lenr + 7;
                                end
                            end
                    end
                end
                Send_Buffer_1(lenS_1:lenS_1+lenr-1) = [recv_package_1(1:lenr-1),102];           % 前提：lenS更新速度比当前更新快

            case 4                                               % normal communication between all Hosts
                for k=1:len_
                    switch Rx_1_data(7*k-3)
                        case 103                                % Handshake ask --> send answer
                            check = check_X(104, Address, Send_Buffer_2);
                            if ((Rx_1_data(7*k-5) ~= 0) && (Rx_1_data(7*k-4) == 0) && ~Handshake_1 && ~check)
                                Address_1 = Rx_1_data(7*k-5);
                                Send_Buffer_2(lenS_2:lenS_2+7) = [Address, Address_1, 104, zeros(1,4), 102];
                            end
                        case 105                                % Delay ask --> send answer
                            check = check_X(106, Address, Send_Buffer_2);
                            if (isequal(Rx_1_data(7*k-5:7*k-4),[Address_1, Address]) && Handshake_1 && ~check) % check Sender & Receiver
                                Send_Buffer_2(lenS_2:lenS_2+7) = [Address, 0, 106, zeros(1,4), 102];
                            end
                        case 107
                            if ((isequal(Rx_1_data(7*k-5),Rx_1_data(7*k-4))) && (Rx_1_data(7*k-5) ~= Address))
                                check = check_Y(Rx_1_data(7*k-5:7*k), recv_package_1) && check_Y(Rx_1_data(7*k-5:7*k), Send_Buffer_1);
                                if ~check
                                    recv_package_1(lenr:lenr+6) = Rx_1_data(7*k-5:7*k+1)';
                                    lenr = lenr + 7;
                                end
                            end
                        otherwise
                            if ((Rx_1_data(7*k-5) ~= Address) && (Rx_1_data(7*k-4) == Address))   % Datablock sent to me --> store in Recv_Buffer
                                check = check_Y(Rx_1_data(7*k-5:7*k), Recv_Buffer');
                                if ~check
                                    Recv_Buffer(lenR+1,:) = Rx_1_data(7*k-5:7*k+1);
                                end
                            elseif ((Rx_1_data(7*k-5) ~=Address) && (Rx_1_data(7*k-4) == 255))    % Datablock is as a Broadcast --> store in Recv_Buffer && Send_Buffer_1
                                check = check_Y(Rx_1_data(7*k-5:7*k), Recv_Buffer');
                                if ~check
                                    Recv_Buffer(lenR+1,:) = Rx_1_data(7*k-5:7*k+1);                          % 可能存在问题，不确定lenR和本程序的更新频率
                                end
                                check = check_Y(Rx_1_data(7*k-5:7*k), recv_package_1) && check_Y(Rx_1_data(7*k-5:7*k), Send_Buffer_1);
                                if ~check
                                    recv_package_1(lenr:lenr+6) = Rx_1_data(7*k-5:7*k+1)';
                                    lenr = lenr + 7;
                                end
                            elseif ((Rx_1_data(7*k-4) ~= Address) && (Rx_1_data(7*k-4) ~= 255))   % Datablock not sent to me --> to transmmit --> store in Send_Buffer_1
                                check = check_Y(Rx_1_data(7*k-5:7*k), recv_package_1) && check_Y(Rx_1_data(7*k-5:7*k), Send_Buffer_1);
                                if ~check
                                    recv_package_1(lenr:lenr+6) = Rx_1_data(7*k-5:7*k+1)';
                                    lenr = lenr + 7;
                                end
                            end
                    end
                end
                Send_Buffer_1(lenS_1:lenS_1+lenr-1) = [recv_package_1(1:lenr-1),102];
        end
	elseif mod_ ~= 0
        fprintf("Eroor: Package length not avalueable!");
	end
end

end

function y = check_X(CMD, adr, Data)          % y: boolean; x: double, [1x100];

x = find(Data==CMD);
y = (~isempty(x));

if y
    y = y && (Data(1,x(1)-2) == adr);
end

end

function y = check_Y(data, Data)          % y: boolean; data: double, [1x6];

x = find(Data==data(3));
y = (~isempty(x));
if y
    for i=1:length(x)
        if(isequal(Data(x(i)-2:x(i)+3),data'))
            y = true;
            break
        else
            y = false;
        end
    end
end

end
